simulink model "main"  (R2018a)
settings: Solver=FixedStepAuto  StartTime=0.0  StopTime=50  FixedStep=0.1  RelTol=1e-3
values from neighbouring files (symbols this model uses):
  A = [0.4126 0 -0.0196;0.0333 0.5207 -0.0413;-0.0101 0 0.2571]    [obsCtrb.m]    (also in trackingScript.m)
  B = [-1.7734 0.0696 0.0734;0.0928 0.4658 0.1051;-0.0424 -0.093 2.0752]    [obsCtrb.m]    (also in trackingScript.m)
  C = eye(3)    [obsCtrb.m]    (also in trackingScript.m)
  K1 = K(1:3,1:3)    [trackingScript.m]
  K2 = K(1:3,4:6)    [trackingScript.m]
settings Model: Creator=Haydar  LastModifiedBy=Haydar

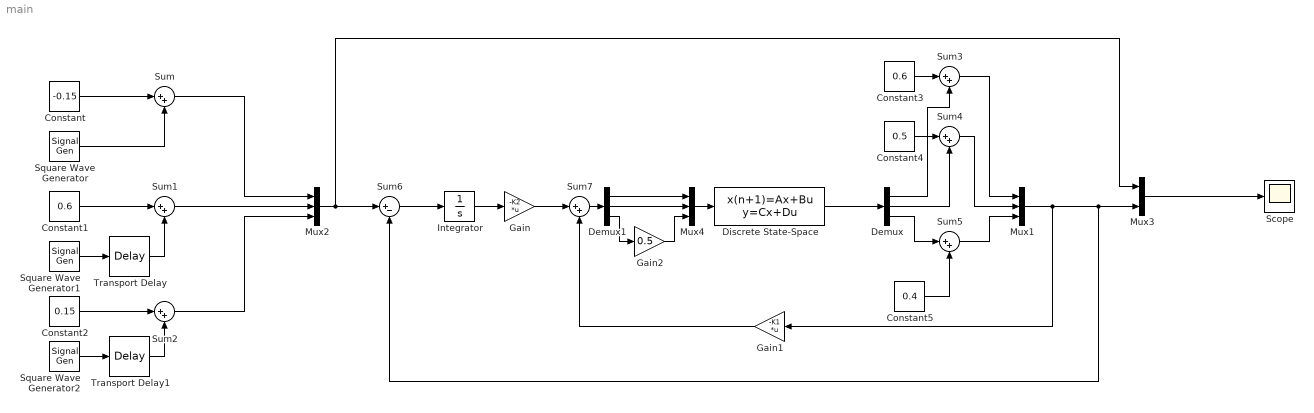
== system main ==
  Constant : Constant  Value=-0.15
  Constant1 : Constant  Value=0.6
  Constant2 : Constant  Value=0.15
  Constant3 : Constant  Value=0.6
  Constant4 : Constant  Value=0.5
  Constant5 : Constant  Value=0.4
  Demux : Demux  Outputs=3
  Demux1 : Demux  Outputs=3
  Discrete State-Space : DiscreteStateSpace  A=A  B=B  C=C  D=zeros(3,3)  SampleTime=0.1
  Gain : Gain  Gain=-K2  Multiplication=Matrix(K*u)
  Gain1 : Gain  Gain=-K1  Multiplication=Matrix(K*u)
  Gain2 : Gain  Gain=0.5
  Integrator : Integrator
  Mux1 : Mux  Inputs=3
  Mux2 : Mux  Inputs=3
  Mux3 : Mux  Inputs=2
  Mux4 : Mux  Inputs=3
  Scope : Scope
  Square Wave Generator : SignalGenerator  WaveForm=square  Amplitude=0.05  Frequency=0.1
  Square Wave Generator1 : SignalGenerator  WaveForm=square  Amplitude=0.1  Frequency=0.1
  Square Wave Generator2 : SignalGenerator  WaveForm=square  Amplitude=0.05  Frequency=0.1
  Sum{,1..5,7} (7 alike) : Sum  Inputs=|++
  Sum6 : Sum  Inputs=|+-
  Transport Delay : TransportDelay  DelayTime=2
  Transport Delay1 : TransportDelay  DelayTime=4
  wires:
  Integrator/1 -> Gain/1
  Square Wave Generator/1 -> Sum/2
  Square Wave Generator2/1 -> Transport Delay1/1
  Constant/1 -> Sum/1
  Constant2/1 -> Sum2/1
  Constant1/1 -> Sum1/1
  Square Wave Generator1/1 -> Transport Delay/1
  Transport Delay/1 -> Sum1/2
  Transport Delay1/1 -> Sum2/2
  Discrete State-Space/1 -> Demux/1
  Constant3/1 -> Sum3/1
  Constant4/1 -> Sum4/1
  Constant5/1 -> Sum5/2
  Demux/1 -> Sum3/2
  Demux/2 -> Sum4/2
  Demux/3 -> Sum5/1
  Sum3/1 -> Mux1/1
  Sum4/1 -> Mux1/2
  Sum5/1 -> Mux1/3
  Mux1/1 -> Gain1/1, Mux3/2, Sum6/2
  Sum6/1 -> Integrator/1
  Gain/1 -> Sum7/1
  Gain1/1 -> Sum7/2
  Sum/1 -> Mux2/1
  Sum1/1 -> Mux2/2
  Sum2/1 -> Mux2/3
  Mux3/1 -> Scope/1
  Mux2/1 -> Mux3/1, Sum6/1
  Sum7/1 -> Demux1/1
  Demux1/3 -> Gain2/1
  Mux4/1 -> Discrete State-Space/1
  Demux1/1 -> Mux4/1
  Demux1/2 -> Mux4/2
  Gain2/1 -> Mux4/3
